simulink model "Dynamics_SIM_EST"  (R2025b)
settings: Solver=FixedStepAuto  StartTime=0.0  StopTime=tspan  FixedStep=dt_sim  RelTol=rel_tol  AbsTol=abs_tol
undefined symbols (not defined in the file): const_voltage, FT_list_test
settings Model: SimulationMode=accelerator  Creator=koryh  LastModifiedBy=rubystanton
settings DataIOCC: ExternalInput=inputStructure  LoadExternalInput=on

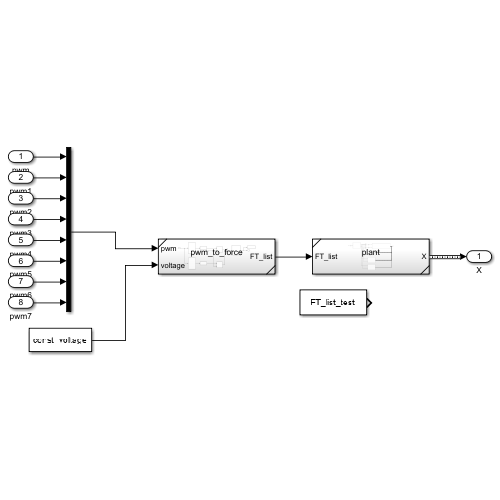
[thumbnail: Simulink's stored preview of the top-level diagram]
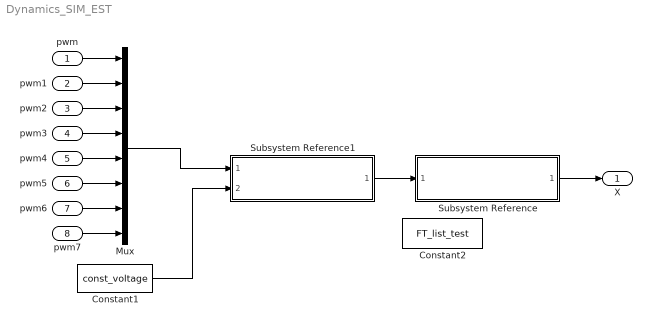
== system Dynamics_SIM_EST ==
  pwm : Inport
  pwm1 : Inport  Port=2
  pwm2 : Inport  Port=3
  pwm3 : Inport  Port=4
  pwm4 : Inport  Port=5
  pwm5 : Inport  Port=6
  pwm6 : Inport  Port=7
  pwm7 : Inport  Port=8
  Constant1 : Constant  Value=const_voltage
  Constant2 : Constant  Value=FT_list_test
  Mux : Mux  Inputs=8
  Subsystem Reference : Subsystem  ReferencedSubsystem=plant
  Subsystem Reference1 : Subsystem  ReferencedSubsystem=pwm_to_force
  X : Outport
  wires:
  Subsystem Reference1/1 -> Subsystem Reference/1
  Constant1/1 -> Subsystem Reference1/2
  Mux/1 -> Subsystem Reference1/1
  Subsystem Reference/1 -> X/1
  pwm/1 -> Mux/1
  pwm1/1 -> Mux/2
  pwm2/1 -> Mux/3
  pwm3/1 -> Mux/4
  pwm4/1 -> Mux/5
  pwm5/1 -> Mux/6
  pwm6/1 -> Mux/7
  pwm7/1 -> Mux/8
